simulink model "SUL_sim_01"  (R2016b)
settings: Solver=VariableStepAuto  StartTime=0.0  StopTime=10.0  RelTol=1e-3
values from neighbouring files (symbols this model uses):
  A = [-L(1)*cos(theta) L(1)*sin(theta)]    [SUL_01.m]
settings Model: Creator=Adam  LastModifiedBy=Adam

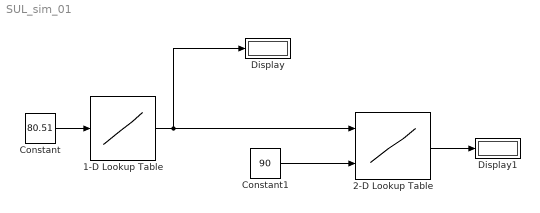
== system SUL_sim_01 ==
  1-D Lookup Table : Lookup_n-D  NumberOfTableDimensions=1  BreakpointsForDimension1=A(:,2)'  Table=[50:10:850]  InternalRulePriority=Speed  RndMeth=Simplest  InputSameDT=on
  2-D Lookup Table : Lookup_n-D  BreakpointsForDimension1=[50:10:850]  BreakpointsForDimension2=[50:5:100]  Table=F'  InternalRulePriority=Speed  RndMeth=Simplest  InputSameDT=on
  Constant : Constant  Value=80.51
  Constant1 : Constant  Value=90
  Display : Display
  Display1 : Display
  wires:
  Constant/1 -> 1-D Lookup Table/1
  1-D Lookup Table/1 -> 2-D Lookup Table/1, Display/1
  Constant1/1 -> 2-D Lookup Table/2
  2-D Lookup Table/1 -> Display1/1
